simulink model "goal"  (R2019a)
settings: Solver=VariableStepAuto  StartTime=0.0  StopTime=10.0  RelTol=1e-3
libraries: simulink x1
settings Model: Creator=jacoboffersen  LastModifiedBy=jacoboffersen

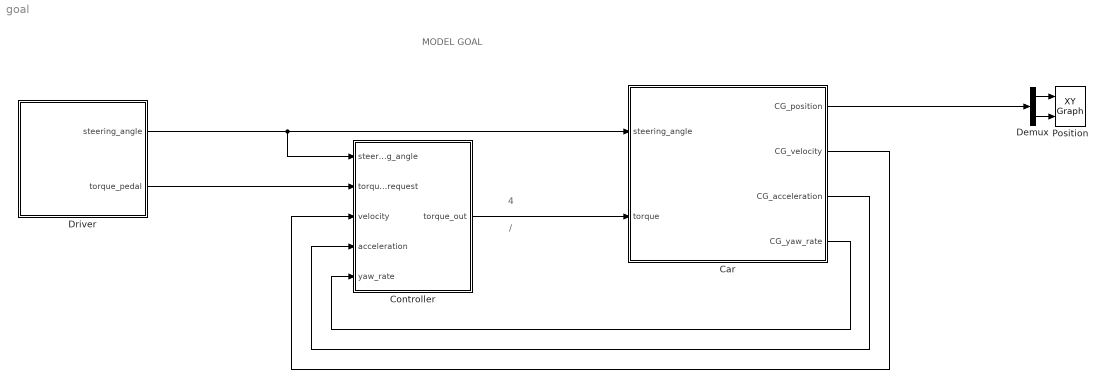
== system goal ==
  note: 4
  note: /
  note: MODEL GOAL
  Car : Subsystem
  Controller : Subsystem
  Demux : Demux  Outputs=2
  Driver : Subsystem
  Position : simulink/Sinks/XY Graph  xmin=-1  xmax=1  ymin=-1  ymax=1  st=-1
  wires:
  Controller/1(torque_out) -> Car/2(torque)
  Car/4(CG_yaw_rate) -> Controller/5(yaw_rate)
  Car/3(CG_acceleration) -> Controller/4(acceleration)
  Car/2(CG_velocity) -> Controller/3(velocity)
  Driver/1(steering_angle) -> Controller/1(steering_angle), Car/1(steering_angle)
  Driver/2(torque_pedal) -> Controller/2(torque_request)
  Demux/2 -> Position/2
  Demux/1 -> Position/1
  Car/1(CG_position) -> Demux/1

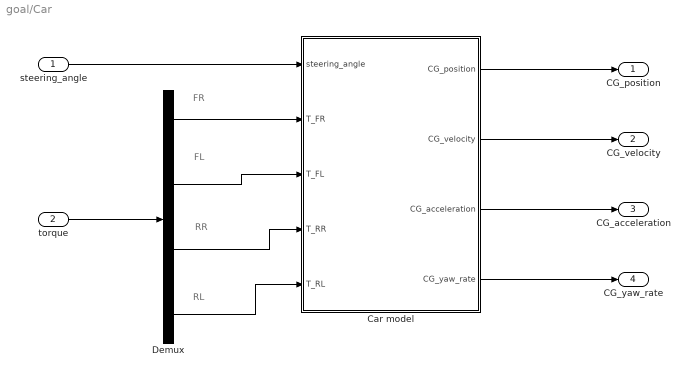
== system goal/Car ==
  note: RL
  note: RR
  note: FL
  note: FR
  steering_angle : Inport
  torque : Inport  Port=2
  Car model : Subsystem
  Demux : Demux
  CG_position : Outport
  CG_velocity : Outport  Port=2
  CG_acceleration : Outport  Port=3
  CG_yaw_rate : Outport  Port=4
  wires:
  torque/1 -> Demux/1
  Demux/1 -> Car model/2(T_FR)
  Demux/2 -> Car model/3(T_FL)
  Demux/3 -> Car model/4(T_RR)
  Demux/4 -> Car model/5(T_RL)
  Car model/1(CG_position) -> CG_position/1
  Car model/4(CG_yaw_rate) -> CG_yaw_rate/1
  Car model/3(CG_acceleration) -> CG_acceleration/1
  Car model/2(CG_velocity) -> CG_velocity/1
  steering_angle/1 -> Car model/1(steering_angle)

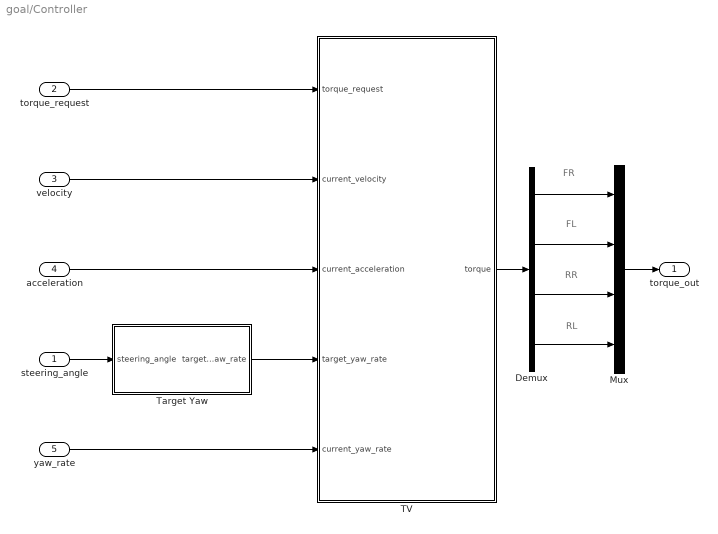
== system goal/Controller ==
  note: FR
  note: RL
  note: FL
  note: RR
  steering_angle : Inport
  torque_request : Inport  Port=2
  velocity : Inport  Port=3
  acceleration : Inport  Port=4
  yaw_rate : Inport  Port=5
  Demux : Demux
  Mux : Mux
  TV : Subsystem
  Target Yaw : Subsystem
  torque_out : Outport
  wires:
  Mux/1 -> torque_out/1
  Demux/1 -> Mux/1
  Demux/2 -> Mux/2
  Demux/3 -> Mux/3
  Demux/4 -> Mux/4
  steering_angle/1 -> Target Yaw/1(steering_angle)
  torque_request/1 -> TV/1(torque_request)
  velocity/1 -> TV/2(current_velocity)
  acceleration/1 -> TV/3(current_acceleration)
  Target Yaw/1(target_yaw_rate) -> TV/4(target_yaw_rate)
  TV/1(torque) -> Demux/1
  yaw_rate/1 -> TV/5(current_yaw_rate)

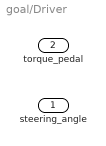
== system goal/Driver ==
  steering_angle : Outport
  torque_pedal : Outport  Port=2

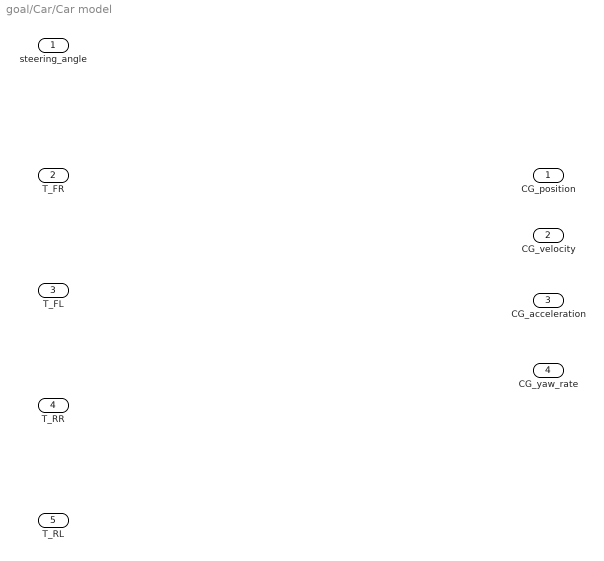
== system goal/Car/Car model ==
  steering_angle : Inport
  T_FR : Inport  Port=2
  T_FL : Inport  Port=3
  T_RR : Inport  Port=4
  T_RL : Inport  Port=5
  CG_position : Outport
  CG_velocity : Outport  Port=2
  CG_acceleration : Outport  Port=3
  CG_yaw_rate : Outport  Port=4

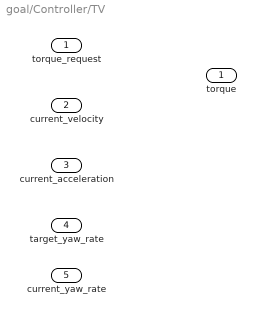
== system goal/Controller/TV ==
  torque_request : Inport
  current_velocity : Inport  Port=2
  current_acceleration : Inport  Port=3
  target_yaw_rate : Inport  Port=4
  current_yaw_rate : Inport  Port=5
  torque : Outport

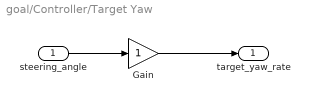
== system goal/Controller/Target Yaw ==
  steering_angle : Inport
  Gain : Gain
  target_yaw_rate : Outport
  wires:
  steering_angle/1 -> Gain/1
  Gain/1 -> target_yaw_rate/1
